simulink model "ODE_Simulink"  (R2015b)
settings: Solver=ode1  StartTime=0.0  StopTime=10.0  FixedStep=0.01  RelTol=1e-3
settings Model: Creator=aemili  LastModifiedBy=aemili

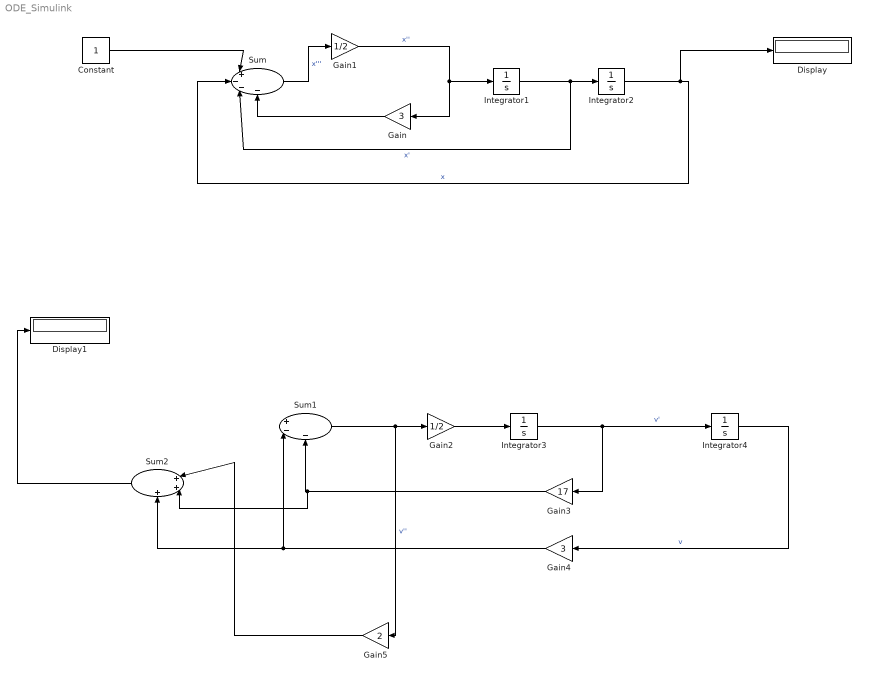
== system ODE_Simulink ==
  Constant : Constant
  Display : Display
  Display1 : Display
  Gain : Gain  Gain=3
  Gain1 : Gain  Gain=1/2
  Gain2 : Gain  Gain=1/2
  Gain3 : Gain  Gain=17
  Gain4 : Gain  Gain=3
  Gain5 : Gain  Gain=2
  Integrator1 : Integrator  InitialCondition=2
  Integrator2 : Integrator  InitialCondition=1
  Integrator3 : Integrator  InitialCondition=2
  Integrator4 : Integrator  InitialCondition=2
  Sum : Sum  Inputs=|+---
  Sum1 : Sum  Inputs=|+--
  Sum2 : Sum  Inputs=|+++
  wires:
  Sum/1 -> Gain1/1  "x'''"
  Integrator1/1 -> Sum/3, Integrator2/1  "x'"
  Integrator2/1 -> Display/1, Sum/2  "x"
  Constant/1 -> Sum/1
  Gain1/1 -> Gain/1, Integrator1/1  "x''"
  Gain/1 -> Sum/4
  Sum1/1 -> Gain5/1, Gain2/1  "v''"
  Gain2/1 -> Integrator3/1
  Integrator3/1 -> Gain3/1, Integrator4/1  "v'"
  Integrator4/1 -> Gain4/1  "v"
  Gain3/1 -> Sum2/2, Sum1/3
  Gain4/1 -> Sum2/3, Sum1/2
  Gain5/1 -> Sum2/1
  Sum2/1 -> Display1/1
